simulink model "SG__MDL_DMA"  (R2022b)
settings: Solver=FixedStepAuto  StartTime=0.0  StopTime=30  FixedStep=50e-6  RelTol=1e-3  EnableMultiTasking=on
model workspace (MAT data in the model file):
  freq_sine = 1000
  src_gain = Simulink.Parameter
  src_gain.Value = 2
  src_gain.DataType = 'auto'
  src_gain.Complexity = 'real'
  src_gain.Dimensions = [1 1]
undefined symbols (not defined in the file or in its folder): N_trig
libraries: speedgoatlib_IO135 x3, simulink x3
settings Model: SimulationMode=external  DataflowThreadingImplementation=Pthreads  Creator=padlewsk  LastModifiedBy=padlewsk
settings SolverCC: ConcurrentTasks=on  AlgebraicLoopSolver=TrustRegion  PositivePriorityOrder=on  AutoInsertRateTranBlk=on
settings DataIOCC: SaveFormat=StructureWithTime
settings OptimizationCC: GainParamInheritBuiltInType=on  UseFloatMulNetSlope=on  RollThreshold=9  EfficientFloat2IntCast=on  SimCompilerOptimization=on
settings DebuggingCC: ReadBeforeWriteMsg=DisableAll  WriteAfterWriteMsg=DisableAll  WriteAfterReadMsg=DisableAll  TasksWithSamePriorityMsg=none  UnconnectedInputMsg=warning  UnconnectedOutputMsg=warning  UnconnectedLineMsg=warning  ModelReferenceSymbolNameMessage=none
settings HardwareCC: ProdBitPerLong=64  ProdLongLongMode=on  ProdHWDeviceType=Intel->x86-64 (Linux 64)
settings ModelReferenceCC: UpdateModelReferenceTargets=IfOutOfDate  EnableRefExpFcnMdlSchedulingChecks=on
settings SFSimCC: SFSimEcho=off
settings RTWCC: Description=Simulink Real-Time  SystemTargetFile=slrealtime.tlc  TemplateMakefile=slrealtime_default_tmf  Toolchain=Simulink Real-Time Toolchain  BuildConfiguration=Faster Runs  CodeExecutionProfiling=on  TargetLang=C++
settings SimulinkRealTimeTargetCC: UseGCCFastMath=on

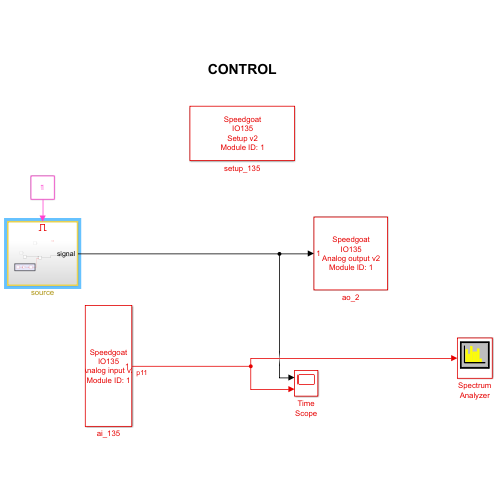
[thumbnail: Simulink's stored preview of the top-level diagram]
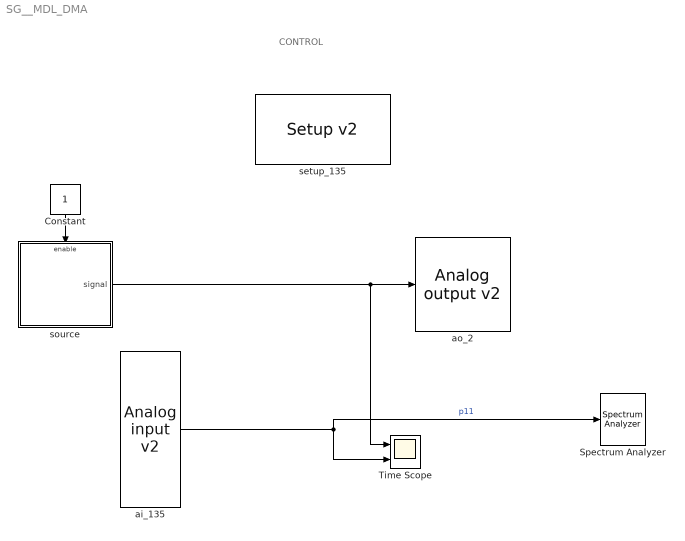
== system SG__MDL_DMA ==
  note: CONTROL
  Constant : Constant
  Spectrum Analyzer : SpectrumAnalyzer
  Time Scope : Scope  NumInputPorts=2
  ai_135 : speedgoatlib_IO135/Analog input v2   parModuleId=1  parSampleTime=-1  parPciSlot=-1  parAdcChannels=1  parAdcVoltageRange=[1 1 1 1]  parAdcOversamplRate=[1 1 1 1]  parAdcContSampling=0  parAdcDmaEnable=0  parAdcActiveDmaDevices=[1 1 1 1]  parAdcFrameSize=1
      settings: SourceProductName=Simulink Real-Time: Speedgoat I/O Blockset
  ao_2 : speedgoatlib_IO135/Analog output v2   parModuleId=1  parSampleTime=-1  parPciSlot=-1  parDacChannels=1  parDacVoltageRange=[4 4 4 4 4 4 4 4 4 4 4 4 4 4 4 4]  parDacInitValues=0  parDacReset=1  parDacSyncOut=1  parDacDmaEnable=0  parDacActiveDmaDevices=[1 1 1 1]  parDacDmaLatency=1  parDacFrameSize=1
      settings: SourceProductName=Simulink Real-Time: Speedgoat I/O Blockset
  setup_135 : speedgoatlib_IO135/Setup v2   parPciSlot=-1  parModuleId=1  parInterModuleSync=None  parConvClockBaseRate=20MHz  parConvClock1Divider=700  parConvClock2Divider=700  parFrameTriggerEnable=off  parFrameTriggerDivider=10  parConvClock1BaseRate=1  parConvClock2BaseRate=1  parFrameTriggerClock=1  parAdcChannels=[1:1]  parAdcRange1=+-5V  parAdcRange2=+-5V  parAdcRange3=+-5V  parAdcRange4=+-5V  parAdcVoltageRange=[1 1 1 1]  parAdcOversampling1=None  parAdcOversampling2=None  parAdcOversampling3=None  parAdcOversampling4=None  parAdcOversamplRate=[1 1 1 1]  parAdcAutoCorrection=on  parAdcContSampling=off  parAdcDmaEnable=off  parAdcDmaClock=Clock 1  parAdcFrameSize_=1  parAdcSampleTime_=-1  parAdcActiveDmaDevices=[1 1 1 1]  parAdcFrameTriggerEnable=0  parAdcFrameSize=1  parAdcSampleTime=3.5e-05  parDacChannels=[1:1]  parDacInitValues=zeros(1,1)  parDacReset=1  parDacRange1=+-5V  parDacRange2=+-5V  parDacRange3=+-5V  parDacRange4=+-5V  parDacRange5=+-5V  parDacRange6=+-5V  parDacRange7=+-5V  parDacRange8=+-5V  parDacRange9=+-5V  parDacRange10=+-5V  parDacRange11=+-5V  parDacRange12=+-5V  parDacRange13=+-5V  parDacRange14=+-5V  parDacRange15=+-5V  parDacRange16=+-5V  parDacVoltageRange=[4 4 4 4 4 4 4 4 4 4 4 4 4 4 4 4]  parDacAutoCorrection=on  parDacSyncOut=on  parDacDmaEnable=off  parDacDmaLatency=As small as possible  parDacDmaClock=Clock 1  parDacFrameSize_=1  parDacSampleTime_=-1  parDacActiveDmaDevices=[1 1 1 1]  parDacFrameTriggerEnable=0  parDacFrameSize=1  parDacSampleTime=3.5e-05  parDoChannels=[]  parDoInitValues=0  parDoReset=1  parDiChannels=[]  parDiDebounceEnable=off  parDiDebounceTime=0  parDiDebounceValue=0  parDioPullRefFront=Pull-up 3.3V  parDioPullRefRear=Floating
      settings: SourceProductName=Simulink Real-Time: Speedgoat I/O Blockset
  source : Subsystem  TreatAsAtomicUnit=on
  wires:
  Constant/1 -> source/Enable
  source/1(signal) -> Time Scope/1, ao_2/1
  ai_135/1 -> Spectrum Analyzer/1, Time Scope/2  "p11"

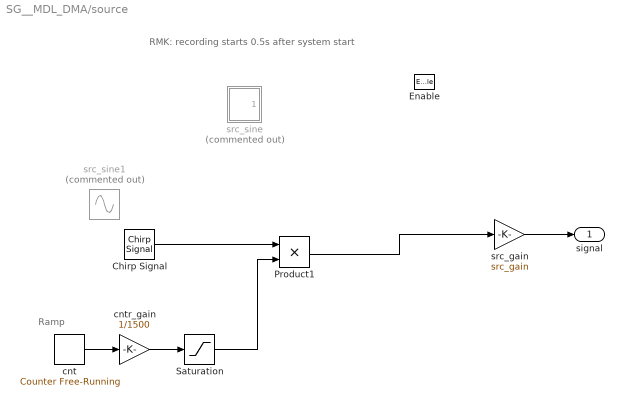
== system SG__MDL_DMA/source ==
  note: RMK: recording starts 0.5s after system start
  note: Ramp
  Enable : EnablePort  StatesWhenEnabling=reset
  Chirp Signal : simulink/Sources/Chirp Signal  f1=100  T=30  f2=350
  Product1 : Product
  Saturation : Saturate  UpperLimit=1  LowerLimit=0
  cnt : simulink/Sources/Counter Free-Running  NumBits=32  tsamp=-1
  cntr_gain : Gain  Gain=1/1500  ParamDataTypeStr=double
  src_gain : Gain  Gain=src_gain
  src_sine : Subsystem  Commented=on
  src_sine1 : Sin  Commented=on  Frequency=freq_sine*2*pi
  signal : Outport  OutputWhenDisabled=reset  InitialOutput=0  VectorParamsAs1DForOutWhenUnconnected=off
  wires:
  src_gain/1 -> signal/1
  Saturation/1 -> Product1/2
  cnt/1 -> cntr_gain/1
  cntr_gain/1 -> Saturation/1
  Product1/1 -> src_gain/1
  Chirp Signal/1 -> Product1/1

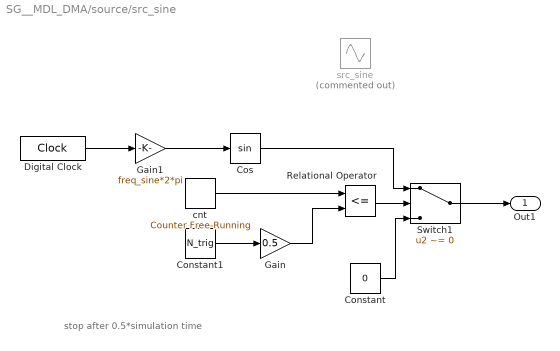
== system SG__MDL_DMA/source/src_sine ==
  note: stop after 0.5*simulation time
  Constant : Constant  Value=0
  Constant1 : Constant  Value=N_trig  VectorParams1D=off  SampleTime=-1
  Cos : Trigonometry
  Digital Clock : DigitalClock  SampleTime=-1
  Gain : Gain  Gain=0.5
  Gain1 : Gain  Gain=freq_sine*2*pi
  Relational Operator : RelationalOperator  Operator=<=  OutDataTypeStr=boolean  RndMeth=Simplest  InputSameDT=off
  Switch1 : Switch  Criteria=u2 ~= 0  SaturateOnIntegerOverflow=off  InputSameDT=off
  cnt : simulink/Sources/Counter Free-Running  NumBits=32  tsamp=-1
  src_sine : Sin  Commented=on  Frequency=freq_sine*2*pi
  Out1 : Outport
  wires:
  Switch1/1 -> Out1/1
  Constant1/1 -> Gain/1
  Relational Operator/1 -> Switch1/2
  cnt/1 -> Relational Operator/1
  Constant/1 -> Switch1/3
  Gain/1 -> Relational Operator/2
  Digital Clock/1 -> Gain1/1
  Gain1/1 -> Cos/1
  Cos/1 -> Switch1/1
